simulink model "Microgrid_w_BESS_Q3_1"  (R2024b)
settings: Solver=VariableStepAuto  StartTime=0.0  StopTime=4  RelTol=1e-3
undefined symbols (not defined in the file): DiscIntNeverNeededParam, ini_SoC, Ion, Lithium, Ts, Ts_Control
libraries: simulink x5, ee_lib x5, spsParallelRLCBranchLib x4, nesl_utility x4, spsCurrentVoltageSimscapeInterfaceLib x3, powerlib_extras x3, spsThreePhaseVIMeasurementLib x2, spsSeriesRLCBranchLib x2, spsMultimeterLib x2, spsThreePhaseSeriesRLCBranchLib x2, spsGroundLib x2, slpidlib x2
(part 2 of 2)

== matlab function Microgrid_w_BESS_Q3_1/Scopes/SoC/MATLAB Function1 ==
  settings: updateMethod=DISCRETE
  data: I_batt input; SoC output; V_batt input; initial_SOC input; Q_nom input; time_scale input; Ts input
function SoC = soc_estimation_with_voltage(I_batt, V_batt, initial_SOC, Q_nom, time_scale, Ts)
%#codegen
% Persistent integrator state
persistent integral_charge SoC_coulomb_state
if isempty(integral_charge)
    integral_charge = 0;
    SoC_coulomb_state = initial_SOC;
end

% Time-scaled charge integration (Ah)
delta_charge = (I_batt * Ts) / 3600; % Positive I_batt means charging
integral_charge = integral_charge + delta_charge * time_scale;

% Update Coulomb-based SoC cumulatively
SoC_coulomb_state = SoC_coulomb_state + (delta_charge * time_scale) / Q_nom;

% Clamp internal state (to prevent runaway)
SoC_coulomb_state = max(0, min(0.9, SoC_coulomb_state));
SoC_coulomb = SoC_coulomb_state;

% Voltage-based correction
V_corr = V_batt - I_batt * 0.1; % R_int = 0.1 Ohm
V_ocv_base = 380 + 50 * SoC_coulomb - 5 * SoC_coulomb^2;
SoC_voltage = max(0, min(1, (V_corr - 380) / 50));  % Linear approximation

% Weighted average
SoC = 0.98 * SoC_coulomb + 0.02 * SoC_voltage;
SoC = max(0, min(0.9, SoC));

% Debugging
assignin('base', 'integral_charge', integral_charge);
assignin('base', 'delta_charge', delta_charge);
assignin('base', 'I_batt', I_batt);
assignin('base', 'SoC_coulomb', SoC_coulomb);
assignin('base', 'SoC_voltage', SoC_voltage);
assignin('base', 'SoC', SoC);
assignin('base', 'V_batt', V_batt);
assignin('base', 'V_ocv_base', V_ocv_base);
assignin('base', 'V_corr', V_corr);
end
